simulink model "modelo"  (Simulink 5.0)
settings: Solver=ode45  StartTime=0.0  StopTime=100  RelTol=1e-3
values from neighbouring files (symbols this model uses):
  Kd = pid(3)    [simular.m]
  Ki = pid(2)    [simular.m]
  Kp = pid(1)    [simular.m]
  Mp = 0    [simular.m]
  tp = 0    [simular.m]
  tr = 0    [simular.m]
  ts = 0    [simular.m]
  ys = 0    [simular.m]
undefined symbols (not defined in the file or in its folder): den, num
libraries: simulink_extras x1
settings Model: LastModifiedBy=alberto  ExtModeTrigMode=oneshot  ExtModeArmWhenConnect=off  LimitDataPoints=off  BooleanDataType=off

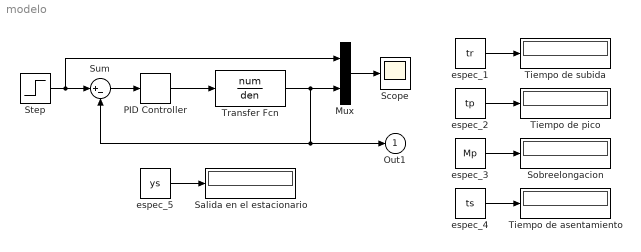
== system modelo ==
  Mux : Mux  Inputs=2
  PID Controller : simulink_extras/Additional Linear/PID Controller  P=Kp  I=Ki  D=Kd
  Salida en el estacionario : Display
  Scope : Scope
      settings: TimeRange=100  YMin=0  YMax=1.4
  Sobreelongacion : Display
  Step : Step  Time=0  SampleTime=0.01
  Sum : Sum  Inputs=|+-  SaturateOnIntegerOverflow=on  InputSameDT=on
  Tiempo de asentamiento : Display
  Tiempo de pico : Display
  Tiempo de subida : Display
  Transfer Fcn : TransferFcn  Numerator=num  Denominator=den
  espec_1 : Constant  Value=tr
  espec_2 : Constant  Value=tp
  espec_3 : Constant  Value=Mp
  espec_4 : Constant  Value=ts
  espec_5 : Constant  Value=ys
  Out1 : Outport
  wires:
  Sum/1 -> PID Controller/1
  Step/1 -> Sum/1, Mux/1
  Mux/1 -> Scope/1
  PID Controller/1 -> Transfer Fcn/1
  Transfer Fcn/1 -> Mux/2, Sum/2, Out1/1
  espec_1/1 -> Tiempo de subida/1
  espec_2/1 -> Tiempo de pico/1
  espec_3/1 -> Sobreelongacion/1
  espec_4/1 -> Tiempo de asentamiento/1
  espec_5/1 -> Salida en el estacionario/1
